simulink model "LoeDetector"  (R2021a)
settings: Solver=FixedStepAuto  StartTime=0.0  StopTime=100  FixedStep=Ts  RelTol=1e-3
InitFcn:
  | LoeDetector_init
values from neighbouring files (symbols this model uses):
  LoeDetectorParams = Simulink.Parameter(loeDetectorParams)    [LoeDetector_init.m]
undefined symbols (not defined in the file or in its folder): loe_detector_filter_sys
settings Model: Creator=bramsvs  LastModifiedBy=root
settings SolverCC: AlgebraicLoopSolver=TrustRegion
settings DataIOCC: ReturnWorkspaceOutputs=off
settings OptimizationCC: DefaultParameterBehavior=Inlined  ZeroExternalMemoryAtStartup=off  ZeroInternalMemoryAtStartup=off
settings DebuggingCC: SFMachineParentedDataDiag=warning  ArithmeticOperatorsInVariantConditions=warning
settings HardwareCC: ProdBitPerPointer=32  ProdBitPerSizeT=32  ProdBitPerPtrDiffT=32  ProdLargestAtomicFloat=None  ProdWordSize=32  ProdLongLongMode=on  ProdHWDeviceType=Custom  TargetLongLongMode=on  TargetIntDivRoundTo=Zero  TargetEndianess=LittleEndian  TargetHWDeviceType=Custom Processor->Custom Processor
settings SFSimCC: CustomCodeUndefinedFunction=UseInterfaceOnly  SimTargetLang=C++
settings RTWCC: Description=Generic Real-Time Target  GenCodeOnly=on  PackageGeneratedCodeAndArtifacts=on  TargetLang=C++
settings CodeAppCC: MATLABSourceComments=on
settings GRTTargetCC: TargetLangStandard=C++03 (ISO)  UtilityFuncGeneration=Shared location  MatFileLogging=off  CodeInterfacePackaging=C++ class  SupportVariableSizeSignals=on

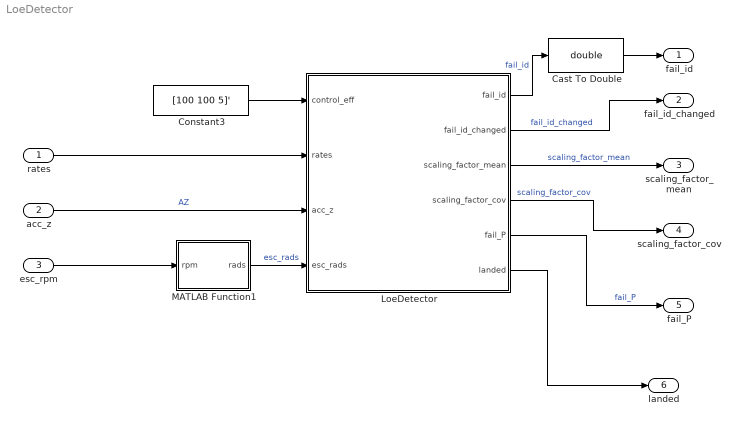
== system LoeDetector ==
  rates : Inport  OutDataTypeStr=double  Unit=rad/s  PortDimensions=3
  acc_z : Inport  Port=2  OutDataTypeStr=double  Unit=m/s^2  PortDimensions=1  LockScale=on
  esc_rpm : Inport  Port=3  OutDataTypeStr=double  PortDimensions=4
  Cast To Double : DataTypeConversion  OutDataTypeStr=double
  Constant3 : Constant  Value=[100 100 5]'
  LoeDetector : MATLAB Function  TreatAsAtomicUnit=on
  MATLAB Function1 : MATLAB Function  TreatAsAtomicUnit=on
  fail_id : Outport  OutDataTypeStr=double  PortDimensions=1  VectorParamsAs1DForOutWhenUnconnected=off
  fail_id_changed : Outport  Port=2  OutDataTypeStr=boolean  VectorParamsAs1DForOutWhenUnconnected=off
  scaling_factor_mean : Outport  Port=3  VectorParamsAs1DForOutWhenUnconnected=off
  scaling_factor_cov : Outport  Port=4  VectorParamsAs1DForOutWhenUnconnected=off
  fail_P : Outport  Port=5  VectorParamsAs1DForOutWhenUnconnected=off
  landed : Outport  Port=6  VectorParamsAs1DForOutWhenUnconnected=off
  wires:
  Constant3/1 -> LoeDetector/1(control_eff)
  LoeDetector/1(fail_id) -> Cast To Double/1  "fail_id"
  rates/1 -> LoeDetector/2(rates)
  acc_z/1 -> LoeDetector/3(acc_z)  "AZ"
  MATLAB Function1/1(rads) -> LoeDetector/4(esc_rads)  "esc_rads"
  esc_rpm/1 -> MATLAB Function1/1(rpm)
  LoeDetector/2(fail_id_changed) -> fail_id_changed/1  "fail_id_changed"
  LoeDetector/4(scaling_factor_cov) -> scaling_factor_cov/1  "scaling_factor_cov"
  LoeDetector/3(scaling_factor_mean) -> scaling_factor_mean/1  "scaling_factor_mean"
  LoeDetector/5(fail_P) -> fail_P/1  "fail_P"
  LoeDetector/6(landed) -> landed/1
  Cast To Double/1 -> fail_id/1

== matlab function LoeDetector/MATLAB Function1 ==
  data: rpm input; rads output
function rads = rpm_to_rads(rpm)

RPM_TO_RADS = 2*pi/60;

rads = RPM_TO_RADS.*rpm;

== matlab function LoeDetector/LoeDetector ==
  data: control_eff input; rates input; acc_z input; esc_rads input; fail_id output; fail_id_changed output; scaling_factor_mean output; scaling_factor_cov output; LoeDetectorParams parameter; loe_detector_filter_sys parameter; fail_P output; landed output
function [fail_id, fail_id_changed, ...
    scaling_factor_mean, scaling_factor_cov, fail_P, landed] = fcn(control_eff, ...
    rates, ...
    acc_z, ...
    esc_rads, ...
    LoeDetectorParams, ... % assigned in `init.m`
loe_detector_filter_sys)

Ts = 1/500; % TODO: to params

n_imu_meas = 3;
n_act = 4;
n_rates = 2; % p, q

% Process and measurement noise
Q = 0.01; % R_1
R = 1; % R_2

persistent landDetector
if isempty(landDetector)
    landDetector = LoeDetectorPkg.LandDetector(800);
end

persistent loeDetector
if isempty(loeDetector)
    loeDetector = LoeDetectorPkg.LoeDetector(loe_detector_filter_sys, ...
        Ts, ...
        n_imu_meas, n_act, n_rates, ...
        Q, R, control_eff, ...
        LoeDetectorParams);
end

persistent changeDetector
if isempty(changeDetector)
    changeDetector = BlocksPkg.ChangeDetector();
end

act_rads_meas = esc_rads';

landed = landDetector.step(act_rads_meas);

[fail_id, log] = loeDetector.step(rates(1:n_rates)', acc_z, act_rads_meas, landed);

[fail_id_changed] = changeDetector.step(fail_id);

scaling_factor_mean = log.scaling_factor_mean;
scaling_factor_cov = log.scaling_factor_cov;
fail_P = log.fail_P;
